simulink model "station2_task"  (Simulink 3.00)
libraries: logiclib x3, mathlib x2, execlib x2, analoglib x1, genlib x1, paramlib x1, speclib x1
settings Model: rev.=3173,  Date=2013-05-31

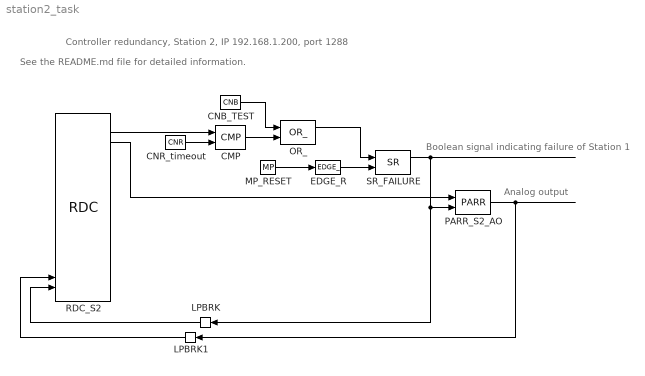
== system station2_task ==
  note: See the README.md file for detailed information.
  note: Controller redundancy, Station 2, IP 192.168.1.200, port 1288
  note: Boolean signal indicating failure of Station 1
  note: Analog output
  CMP : analoglib/CMP  hys=0
  CNB_TEST : mathlib/CNB  YCN=off
  CNR_timeout : mathlib/CNR  ycn=5
  EDGE_R : logiclib/EDGE_  iedge=1: Rising edge
  LPBRK : execlib/LPBRK  Orientation=left
  LPBRK1 : execlib/LPBRK  Orientation=left
  MP_RESET : genlib/MP  pwidth=1  BSTATE=off  RPTF=off
  OR_ : logiclib/OR_
  PARR_S2_AO : paramlib/PARR  par=3.7  SATF=off  hilim=1  lolim=-1
  RDC_S2 : speclib/RDC  target=192.168.1.100  rport=1288  lport=1288  id=1  period=0.5
  SR_FAILURE : logiclib/SR
  wires:
  CMP/1 -> OR_/2
  CNB_TEST/1 -> OR_/1
  CNR_timeout/1 -> CMP/2
  EDGE_R/1 -> SR_FAILURE/2
  LPBRK/1 -> RDC_S2/17
  LPBRK1/1 -> RDC_S2/16
  MP_RESET/1 -> EDGE_R/1
  OR_/1 -> SR_FAILURE/1
  PARR_S2_AO/1 -> LPBRK1/1
  RDC_S2/2 -> CMP/1
  RDC_S2/3 -> PARR_S2_AO/1
  SR_FAILURE/1 -> LPBRK/1, PARR_S2_AO/2
